simulink model "Question6_AkankshaMurali"  (R2023b)
settings: Solver=VariableStepAuto  StartTime=0.0  StopTime=10.0  RelTol=1e-3
settings Model: Creator=akank  LastModifiedBy=akank

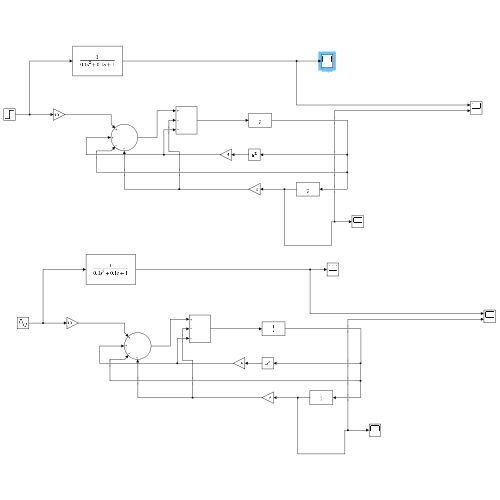
[thumbnail: Simulink's stored preview of the top-level diagram]
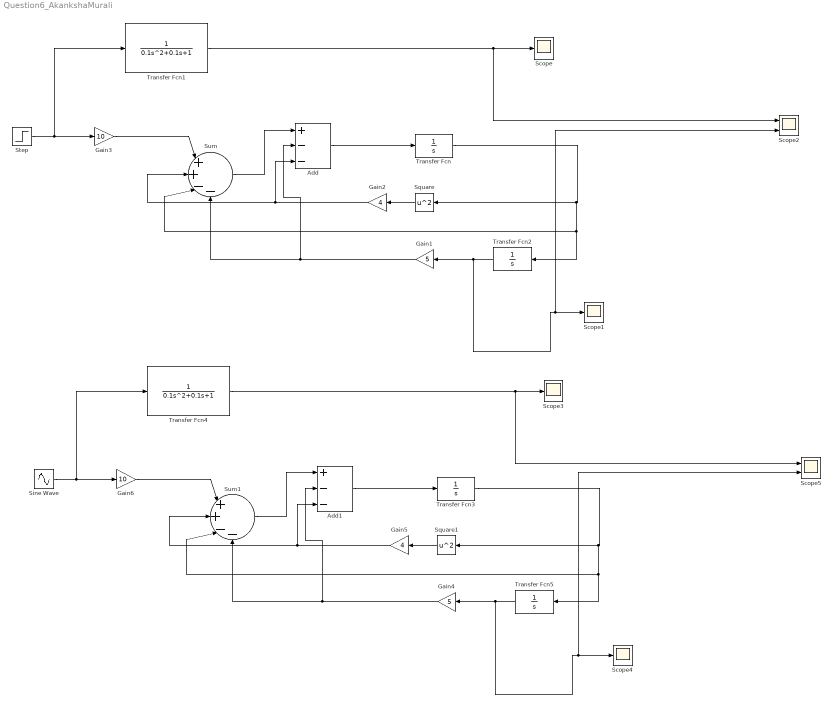
== system Question6_AkankshaMurali ==
  Add : Sum  Inputs=+--
  Add1 : Sum  Inputs=+--
  Gain1 : Gain  Gain=5
  Gain2 : Gain  Gain=4
  Gain3 : Gain  Gain=10
  Gain4 : Gain  Gain=5
  Gain5 : Gain  Gain=4
  Gain6 : Gain  Gain=10
  Scope{,1,3..4} (4 alike) : Scope
  Scope2 : Scope  NumInputPorts=2
  Scope5 : Scope  NumInputPorts=2
  Sine Wave : Sin  SampleTime=0
  Square : Math  Operator=square  OutputSignalType=real
  Square1 : Math  Operator=square  OutputSignalType=real
  Step : Step  SampleTime=0
  Sum : Sum  Inputs=|++--
  Sum1 : Sum  Inputs=|++--
  Transfer Fcn{,2..3,5} (4 alike) : TransferFcn  Denominator=[1 0]
  Transfer Fcn1 : TransferFcn  Denominator=[0.1 0.1 1]
  Transfer Fcn4 : TransferFcn  Denominator=[0.1 0.1 1]
  wires:
  Step/1 -> Transfer Fcn1/1, Gain3/1
  Gain3/1 -> Sum/1
  Transfer Fcn/1 -> Square/1, Transfer Fcn2/1, Sum/3
  Square/1 -> Gain2/1
  Gain1/1 -> Sum/4, Add/2
  Transfer Fcn1/1 -> Scope2/1, Scope/1
  Add/1 -> Transfer Fcn/1
  Gain2/1 -> Sum/2, Add/3
  Transfer Fcn2/1 -> Scope2/2, Scope1/1, Gain1/1
  Sum/1 -> Add/1
  Square1/1 -> Gain5/1
  Gain4/1 -> Sum1/4, Add1/2
  Transfer Fcn3/1 -> Square1/1, Transfer Fcn5/1, Sum1/3
  Sine Wave/1 -> Transfer Fcn4/1, Gain6/1
  Transfer Fcn4/1 -> Scope5/1, Scope3/1
  Add1/1 -> Transfer Fcn3/1
  Gain6/1 -> Sum1/1
  Sum1/1 -> Add1/1
  Transfer Fcn5/1 -> Scope5/2, Scope4/1, Gain4/1
  Gain5/1 -> Sum1/2, Add1/3
